simulink model "model_Ster_Adaptacyjne_2_rzedu"  (R2022a)
settings: Solver=FixedStepAuto  StartTime=0.0  StopTime=100  FixedStep=0.01  RelTol=1e-3
values from neighbouring files (symbols this model uses):
  gamma = gamma_vec(i)    [Modified_MIT_skrypt_Ster_Adaptacyjne_am.m]    (also in skrypt_Ster_Adaptacyjne.m; skrypt_Ster_Adaptacyjne_2_rzedu.m; skrypt_Ster_Adaptacyjne_am.m)
settings Model: Creator=marci  LastModifiedBy=marci

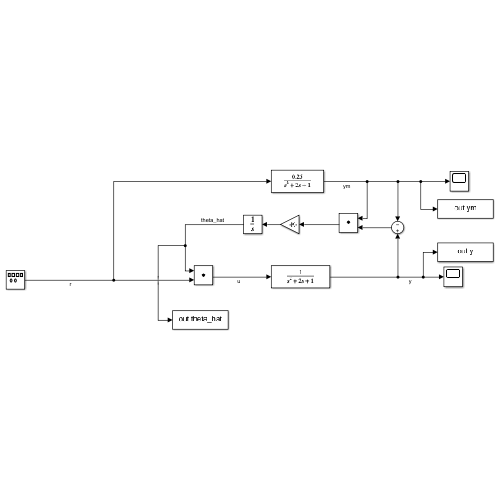
[thumbnail: Simulink's stored preview of the top-level diagram]
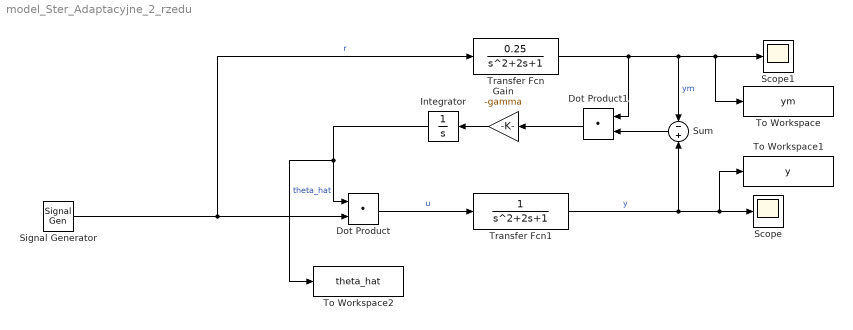
== system model_Ster_Adaptacyjne_2_rzedu ==
  Dot Product : DotProduct  OutDataTypeStr=Inherit: Inherit via internal rule
  Dot Product1 : DotProduct  OutDataTypeStr=Inherit: Inherit via internal rule
  Gain : Gain  Gain=-gamma
  Integrator : Integrator
  Scope : Scope
  Scope1 : Scope
  Signal Generator : SignalGenerator  Frequency=0.1
  Sum : Sum  Inputs=-+
  To Workspace : ToWorkspace  VariableName=ym  SaveFormat=Timeseries  SampleTime=-1
  To Workspace1 : ToWorkspace  VariableName=y  SaveFormat=Timeseries  SampleTime=-1
  To Workspace2 : ToWorkspace  VariableName=theta_hat  SaveFormat=Timeseries  SampleTime=-1
  Transfer Fcn : TransferFcn  Numerator=[0.25]
  Transfer Fcn1 : TransferFcn
  wires:
  Transfer Fcn1/1 -> To Workspace1/1, Scope/1, Sum/2  "y"
  Dot Product1/1 -> Gain/1
  Sum/1 -> Dot Product1/2
  Gain/1 -> Integrator/1
  Transfer Fcn/1 -> To Workspace/1, Scope1/1, Sum/1, Dot Product1/1  "ym"
  Dot Product/1 -> Transfer Fcn1/1  "u"
  Integrator/1 -> To Workspace2/1, Dot Product/1  "theta_hat"
  Signal Generator/1 -> Transfer Fcn/1, Dot Product/2  "r"
